simulink model "bt1"  (R2019a)
settings: Solver=ode5  StartTime=0.0  StopTime=60  FixedStep=0.01  RelTol=1e-3
undefined symbols (not defined in the file): sigbuilder_block
libraries: fuzblock x1
settings Model: Creator=ASUS  LastModifiedBy=ASUS

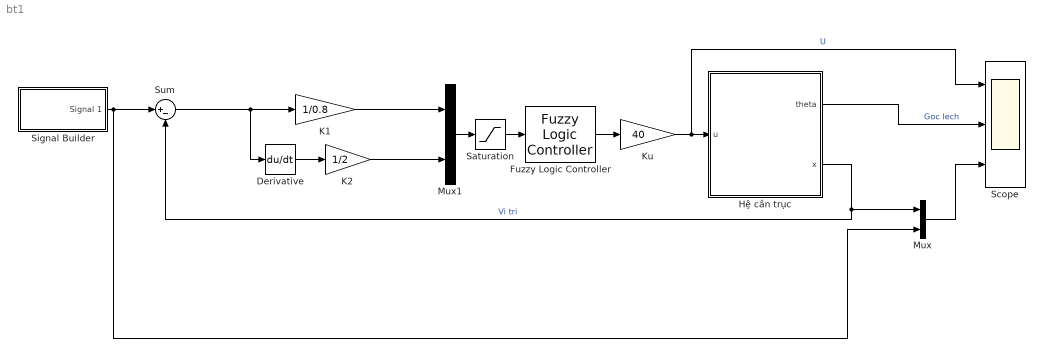
== system bt1 ==
  Derivative : Derivative
  Fuzzy Logic Controller : fuzblock/Fuzzy Logic  Controller  FIS='bt2.fis'  OutputSampleNumber=101  DataType=double  FuzzifiedInputs=off  RuleFiringStrengths=off  RuleOutputs=off  AggregatedOutputs=off  SimulateUsing=Interpreted execution  OutOfRangeInputValueMessage=warning  NoRuleFiredMessage=warning  EmptyOutputFuzzySetMessage=warning
  Hệ cần trục : Subsystem  mask{M=0.5, m_=2, l=0.6, g=9.81}
      mask prompts: m_ "m"
      mask Display: image(imread('bt1.png'))
  K1 : Gain  Gain=1/0.8
  K2 : Gain  Gain=1/2
  Ku : Gain  Gain=40
  Mux : Mux  Inputs=2
  Mux1 : Mux  Inputs=2
  Saturation : Saturate  UpperLimit=1  LowerLimit=-1
  Scope : Scope  NumInputPorts=3
  Signal Builder : Subsystem  Tag=STV Subsys  LoadFcn=sigbuilder_block('load');  StartFcn=sigbuilder_block('start');  StopFcn=sigbuilder_block('stop');  ClipboardFcn=sigbuilder_block('clipboard');  mask(Sigbuilder block){tuvar=[0:10]}
      mask help: Simulink:masks:SigbuilderBlock_MD
      mask init:
      | if ~strcmp(get_param(bdroot(gcbh),'SimulationStatus'),'stopped') tuvar = sigbuilder_block('maskInit'); end
      settings: CopyFcn=sigbuilder_block('copy');  DeleteFcn=sigbuilder_block('delete');  ModelCloseFcn=sigbuilder_block('modelClose');  PreSaveFcn=sigbuilder_block('preSave');  PauseFcn=sigbuilder_block('pause');  ContinueFcn=sigbuilder_block('continue');  NameChangeFcn=sigbuilder_block('namechange');  OpenFcn=sigbuilder_block('open',[558.6 145.8 550.8 400.2 ]);  CloseFcn=sigbuilder_block('close');
      mask Display: plot(0, 0, 100, 100,[2, 2, 32, 32, 2], [68, 8, 8, 68, 68],[32, 2], [38, 38], [32, 19, 2],[53, 60, 44], [32, 17, 17, 2],[16, 16, 31, 31]);txt = getActiveGroup(gcbh);text(2, 100, txt,'verticalAlignment', 'top');
  Sum : Sum  Inputs=|+-
  wires:
  Signal Builder/1(Signal 1) -> Mux/2, Sum/1
  Hệ cần trục/2(x) -> Mux/1, Sum/2  "Vi tri"
  Mux/1 -> Scope/3
  Hệ cần trục/1(theta) -> Scope/2  "Goc lech"
  Derivative/1 -> K2/1
  Mux1/1 -> Saturation/1
  Saturation/1 -> Fuzzy Logic Controller/1
  Fuzzy Logic Controller/1 -> Ku/1
  Sum/1 -> K1/1, Derivative/1
  K2/1 -> Mux1/2
  K1/1 -> Mux1/1
  Ku/1 -> Scope/1, Hệ cần trục/1(u)  "U"

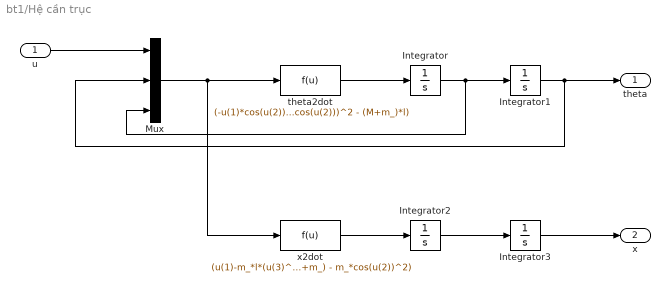
== system bt1/Hệ cần trục ==
  u : Inport
  Integrator{,1..3} (4 alike) : Integrator
  Mux : Mux  Inputs=3
  theta2dot : Fcn  Expr=(-u(1)*cos(u(2))+m_*g*(u(3)^2)*sin(u(2))*cos(u(2))+(M+m_)*g*sin(u(2))) / (m_*l*(cos(u(2)))^2 - (M+m_)*l)
  x2dot : Fcn  Expr=(u(1)-m_*l*(u(3)^2)*sin(u(2)) - m_*g*sin(u(2))*cos(u(2)) ) / ((M+m_) - m_*cos(u(2))^2)
  theta : Outport
  x : Outport  Port=2
  wires:
  u/1 -> Mux/1
  theta2dot/1 -> Integrator/1
  Integrator/1 -> Mux/3, Integrator1/1
  Integrator1/1 -> Mux/2, theta/1
  Mux/1 -> x2dot/1, theta2dot/1
  Integrator3/1 -> x/1
  Integrator2/1 -> Integrator3/1
  x2dot/1 -> Integrator2/1

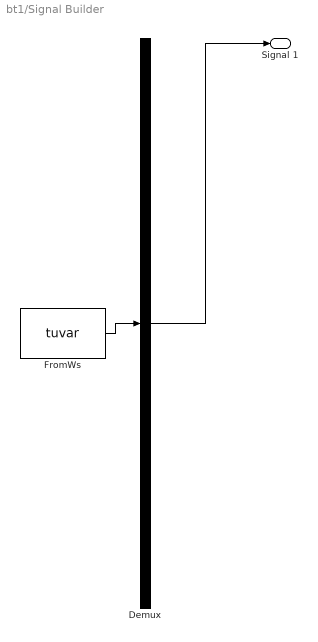
== system bt1/Signal Builder ==
  Demux : Demux  Tag=STV Demux  Outputs=1
  FromWs : FromWorkspace  Tag=STV FromWs  VariableName=tuvar  SampleTime=0
      SigBuilderData=|
      | common.afterFinalStr = 'Extrapolate'
      | common.sampleTime = 0
      | dataSet.timeRange = [0 60]
      | dataSet.name = 'Group 1'
      | sbobj.Groups.Name = 'Group 1'
      | sbobj.Groups.Signals.Name = 'Signal 1'
      | sbobj.Groups.Signals.XData = [0 10 10 20 20 30 30 39.9 39.9 47.2 50 50 60]
      | sbobj.Groups.Signals.YData = [0.45 0.45 0.2 0.2 0.8 0.8 0.55 0.55 0.1 0.1 0.1 0.65 0.65]
      | sbobj.Groups.TimeRange = [0 60]
  Signal 1 : Outport  Tag=STV Outport
  wires:
  Demux/1 -> Signal 1/1
  FromWs/1 -> Demux/1
